simulink library "simpleDragTurbine_ul"  (R2018b)
settings: Solver=VariableStepAuto  StartTime=0.0  StopTime=10.0  RelTol=1e-3
libraries: vrlib x2, eulAng2RotMat_ul x1, dynamicPressure_ul x1, vectorDirection x1
settings Model: Creator=Ayaz  LastModifiedBy=asiddiq2

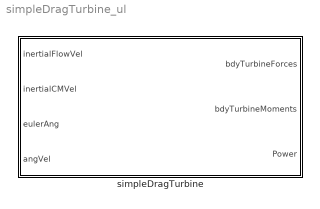
== system simpleDragTurbine_ul ==
  simpleDragTurbine : Subsystem  TreatAsAtomicUnit=on  mask{rhoFluid=1, turbDia=[1 1], turbCp=[0.5 0.5], turbCd=[0.8 0.8], turbPos=[0 -1 0;0 1 0]';}
      mask prompts: rhoFluid "Fluid density"; turbDia "Turbine diameter"; turbCp "Turbine power coefficient"; turbCd "Turbine drag coefficient"; turbPos "Turbine position vector"
      mask TypeOptions rhoFluid: dynamicPressure/rhoFluid
      mask DialogControl ParameterGroupVar Prompt: Environment
      mask DialogControl Container3 Prompt: Turbine
      mask DialogControl Container4 Prompt: Turbine location

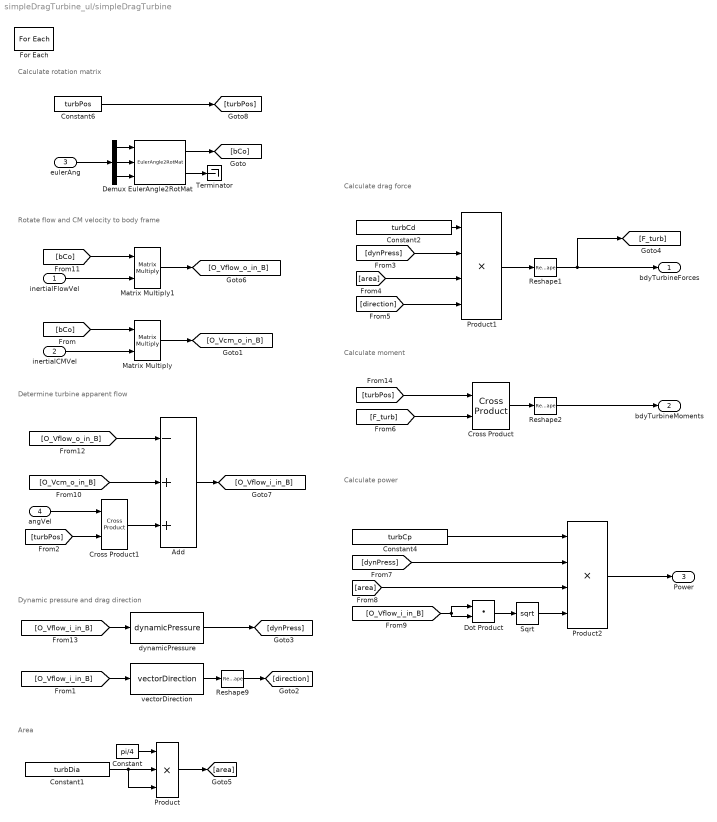
== system simpleDragTurbine_ul/simpleDragTurbine ==
  note: Determine turbine apparent flow
  note: Rotate flow and CM velocity to body frame
  note: Area
  note: Calculate rotation matrix
  note: Calculate drag force
  note: Calculate power
  note: Dynamic pressure and drag direction
  note: Calculate moment
  inertialFlowVel : Inport  PortDimensions=[3,1]
  inertialCMVel : Inport  Port=2  PortDimensions=[3,1]
  eulerAng : Inport  Port=3  PortDimensions=[3,1]
  angVel : Inport  Port=4  PortDimensions=[3,1]
  Add : Sum  Inputs=-++
  Constant : Constant  Value=pi/4
  Constant1 : Constant  Value=turbDia  VectorParams1D=off
  Constant2 : Constant  Value=turbCd  VectorParams1D=off
  Constant4 : Constant  Value=turbCp  VectorParams1D=off
  Constant6 : Constant  Value=turbPos  VectorParams1D=off
  Cross Product : vrlib/Utilities/Cross Product
      settings: SourceProductBaseCode=VR
  Cross Product1 : vrlib/Utilities/Cross Product
      settings: SourceProductBaseCode=VR
  Demux : Demux  Outputs=3
  Dot Product : DotProduct  InputSameDT=on  OutDataTypeStr=Inherit: Inherit via internal rule
  EulerAngle2RotMat : eulAng2RotMat_ul/EulerAngle2RotMat  SystemSampleTime=-1
  For Each : ForEach  DisableCoverage=on  IterateSubsysMaskParameter=off,off,off,off,off  SubsysMaskParameterIterationDimension=1,1,1,1,1  IndexMode=One-based
  Matrix Multiply : Product  Multiplication=Matrix(*)
  Matrix Multiply1 : Product  Multiplication=Matrix(*)
  Product : Product  Inputs=3
  Product1 : Product  Inputs=4
  Product2 : Product  Inputs=4
  Reshape1 : Reshape  OutputDimensionality=Column vector (2-D)
  Reshape2 : Reshape  OutputDimensionality=Column vector (2-D)
  Reshape9 : Reshape  OutputDimensionality=Column vector (2-D)
  Sqrt : Sqrt  SaturateOnIntegerOverflow=on
  Terminator : Terminator
  dynamicPressure : dynamicPressure_ul/dynamicPressure  rhoFluid=rhoFluid
  vectorDirection : vectorDirection/vectorDirection  SystemSampleTime=-1
  bdyTurbineForces : Outport  PortDimensions=[3,1]  ConcatenationDimension=2
  bdyTurbineMoments : Outport  Port=2  PortDimensions=[3,1]  ConcatenationDimension=2
  Power : Outport  Port=3  PortDimensions=[1,1]  ConcatenationDimension=2
  wires:
  inertialCMVel/1 -> Matrix Multiply/2
  inertialFlowVel/1 -> Matrix Multiply1/2
  dynamicPressure/1 -> [dynPress]
  vectorDirection/1 -> Reshape9/1
  [O_Vflow_i_in_B] -> dynamicPressure/1
  EulerAngle2RotMat/2 -> Terminator/1
  eulerAng/1 -> Demux/1
  Demux/3 -> EulerAngle2RotMat/3
  EulerAngle2RotMat/1 -> [bCo]
  Demux/2 -> EulerAngle2RotMat/2
  Demux/1 -> EulerAngle2RotMat/1
  [O_Vflow_i_in_B] -> vectorDirection/1
  Cross Product/1 -> Reshape2/1
  Constant/1 -> Product/1
  Product/1 -> [area]
  Product1/1 -> Reshape1/1
  Reshape9/1 -> [direction]
  Constant1/1 -> Product/3, Product/2
  Constant2/1 -> Product1/1
  [dynPress] -> Product1/2
  [area] -> Product1/3
  [direction] -> Product1/4
  [turbPos] -> Cross Product/1
  [F_turb] -> Cross Product/2
  [area] -> Product2/3
  [dynPress] -> Product2/2
  Constant4/1 -> Product2/1
  [O_Vflow_i_in_B] -> Dot Product/1, Dot Product/2
  Dot Product/1 -> Sqrt/1
  Sqrt/1 -> Product2/4
  Reshape1/1 -> bdyTurbineForces/1, [F_turb]
  Reshape2/1 -> bdyTurbineMoments/1
  [bCo] -> Matrix Multiply/1
  Matrix Multiply/1 -> [O_Vcm_o_in_B]
  [turbPos] -> Cross Product1/2
  angVel/1 -> Cross Product1/1
  Cross Product1/1 -> Add/3
  [O_Vcm_o_in_B] -> Add/2
  [bCo] -> Matrix Multiply1/1
  Matrix Multiply1/1 -> [O_Vflow_o_in_B]
  [O_Vflow_o_in_B] -> Add/1
  Add/1 -> [O_Vflow_i_in_B]
  Constant6/1 -> [turbPos]
  Product2/1 -> Power/1
